simulink model "practical_voltage_source"  (R2017b)
settings: Solver=ode1  StartTime=0.0  StopTime=2e-3  FixedStep=Ts  RelTol=1e-3
PostLoadFcn:
  | , if any(exist('dsrtsu_mdlpostloadfcn', 'file') == [2, 3, 6]), try dsrtsu_mdlpostloadfcn('Execute', bdroot); catch fprintf('Error in PostLoadFcn (dsrtsu_mdlpostloadfcn) for model "%s":\n %s\n', bdroot, lasterr); end, end,
  | init_practical_voltage_source;
values from neighbouring files (symbols this model uses):
  i_L_init = 1    [init_parameters.m]
  v_C_init = 1.1    [init_parameters.m]
undefined symbols (not defined in the file or in its folder): Cf, Lf, RCf, RLf
Description:
  | Standard RTI1005 template.
  | Supported MATLAB version:  R2017b.
settings Model: Tag=RTI1005  DSRTSU_INTERNAL_RTI_VER=540  DSRTSU_INTERNAL_RTI_TYPE=rti1005  RTICANMMDATA=struct('GeneralSetupData',struct('modelroot','C:\Projects\Simulink\PE_1\w3\lec13','generalsettings',struct('filesettings',struct('destfolder',struct('Name','RTICANMM_FILES','Check',1),'buildfolder',struct('Name','.','Check',1),'AbsDestfolder',struct('Name','C:\Projects\Simulink\PE_1\w3\lec13\RTICANMM_FILES'),'AbsBuildfolder',struct('Name','C:\Projects\Simulink\PE_1\w3\lec13'))),'options',struct('addpaths',1,'rmpaths',1,'addtrcexclusion',logical(1),'cannavigator',struct('checkmonitoring',0),'show_usrtrc',0,'use_usrtrc',0),'advanced',struct('options',ones(1,100)),'MPSetup',{{}},'RTI',struct('Type','RTI1005','Ver','7.12','Date','02-May-2019'),'modelname','practical_voltage_source','block','practical_voltage_source'))  DSRTSU_INTERNAL_RTIFPGA=130  Creator=CA72672  LastModifiedBy=CA72672
settings OptimizationCC: BlockReduction=off  OptimizeBlockIOStorage=off  BufferReuse=off  GlobalBufferReuse=off  ExpressionFolding=off  LocalBlockOutputs=off
settings HardwareCC: ProdBitPerPointer=32  ProdBitPerSizeT=32  ProdBitPerPtrDiffT=32  ProdLargestAtomicInteger=Integer  ProdEndianess=BigEndian  ProdWordSize=32  ProdHWDeviceType=Custom Processor->Custom  TargetIntDivRoundTo=Zero  TargetEndianess=BigEndian  TargetHWDeviceType=Custom Processor->Custom
settings SFSimCC: MATLABDynamicMemAlloc=off
settings RTWCC: SystemTargetFile=rti1005.tlc  MakeCommand=make_rti  TemplateMakefile=rti1005.tmf  Description=dSPACE DS1005 Hardware Platform
settings CodeAppCC: StateflowObjectComments=on
settings STFCustomTargetCC: ParMdlRefBuildCompliant=on  MatFileLogging=on  GRTInterface=off  SystemTargetFile=rti1005.tlc
settings GRTTargetCC: TargetLangStandard=C89/C90 (ANSI)  CompOptLevelCompliant=off  ConcurrentExecutionCompliant=off  CombineOutputUpdateFcns=off  CPPClassGenCompliant=off  UseToolchainInfoCompliant=off
settings ConfigComp: CovMetricSettings=dswe

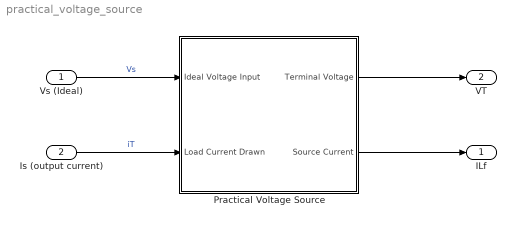
== system practical_voltage_source ==
  Vs (Ideal) : Inport
  Is (output current) : Inport  Port=2
  Practical Voltage Source : Subsystem
  ILf : Outport
  VT : Outport  Port=2
  wires:
  Vs (Ideal)/1 -> Practical Voltage Source/1(Ideal Voltage Input)  "Vs"
  Is (output current)/1 -> Practical Voltage Source/2(Load Current Drawn)  "iT"
  Practical Voltage Source/2(Source Current) -> ILf/1
  Practical Voltage Source/1(Terminal Voltage) -> VT/1

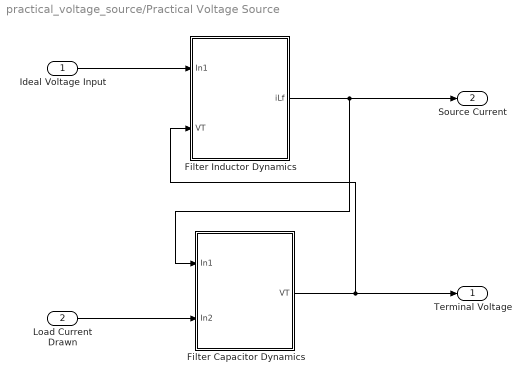
== system practical_voltage_source/Practical Voltage Source ==
  Ideal Voltage Input : Inport
  Load Current Drawn : Inport  Port=2
  Filter Capacitor Dynamics : Subsystem
  Filter Inductor Dynamics : Subsystem
  Terminal Voltage : Outport
  Source Current : Outport  Port=2
  wires:
  Filter Inductor Dynamics/1(iLf) -> Filter Capacitor Dynamics/1(In1), Source Current/1
  Ideal Voltage Input/1 -> Filter Inductor Dynamics/1(In1)
  Filter Capacitor Dynamics/1(VT) -> Filter Inductor Dynamics/2(VT), Terminal Voltage/1
  Load Current Drawn/1 -> Filter Capacitor Dynamics/2(In2)

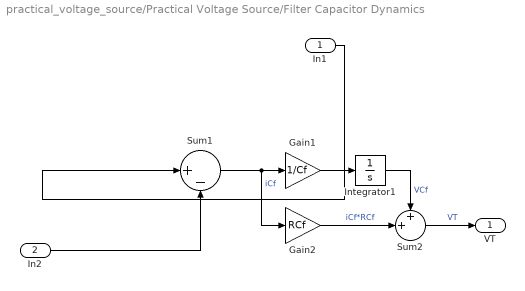
== system practical_voltage_source/Practical Voltage Source/Filter Capacitor Dynamics ==
  In1 : Inport
  In2 : Inport  Port=2
  Gain1 : Gain  Gain=1/Cf
  Gain2 : Gain  Gain=RCf
  Integrator1 : Integrator  InitialCondition=v_C_init
  Sum1 : Sum  Inputs=|+-
  Sum2 : Sum  Inputs=++|
  VT : Outport
  wires:
  In2/1 -> Sum1/2
  Integrator1/1 -> Sum2/1  "VCf"
  Sum1/1 -> Gain2/1, Gain1/1  "iCf"
  Gain2/1 -> Sum2/2  "iCf*RCf"
  Sum2/1 -> VT/1  "VT"
  Gain1/1 -> Integrator1/1
  In1/1 -> Sum1/1

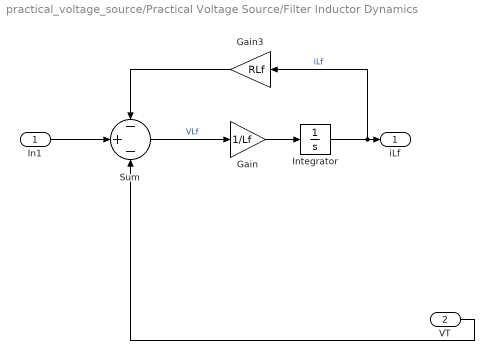
== system practical_voltage_source/Practical Voltage Source/Filter Inductor Dynamics ==
  In1 : Inport
  VT : Inport  Port=2
  Gain : Gain  Gain=1/Lf
  Gain3 : Gain  Gain=RLf
  Integrator : Integrator  InitialCondition=i_L_init
  Sum : Sum  Inputs=-+-
  iLf : Outport
  wires:
  Gain3/1 -> Sum/1
  Sum/1 -> Gain/1  "VLf"
  Gain/1 -> Integrator/1
  Integrator/1 -> Gain3/1, iLf/1  "iLf"
  In1/1 -> Sum/2
  VT/1 -> Sum/3
